simulink model "Ghost"  (Simulink 8.1)
settings: Solver=ode1  StartTime=0.0  StopTime=inf  FixedStep=Ts  MaxStep=1e-3  RelTol=1e-3
PostLoadFcn:
  | NREL_Mode=1; Ghost_init;
InitFcn:
  | NREL_Mode=1; Ghost_init;
values from neighbouring files (symbols this model uses):
  Ts = 100E-6    (= 0.0001)    [BANSHEE_init.m]    (also in Ghost_init.m)
undefined symbols (not defined in the file or in its folder): Stim
libraries: simulink x75, artemis x11, relay_housing_lib x4, rtlab x1, utility_service_lib x1, communications_lib x1, Feeder1_lib x1, Feeder2_lib x1, Feeder3_lib x1, Feeder4_lib x1, powerlib x1
(part 1 of 2)
settings Model: ARTEMISmethode_block_infos=$$__separator__$$Ghost/ARTEMIS Guide$$__separator__$$  Creator=RE25624  LastModifiedBy=pkoralew  BufferReuse=off
settings SolverCC: ZeroCrossAlgorithm=Adaptive
settings DataIOCC: ExternalInput=getinputstruct(op_snapshot1)  InitialState=getstatestruct(op_snapshot1)  LimitDataPoints=off  MaxDataPoints=90060  SignalLoggingSaveFormat=Dataset  SaveOutput=off  SignalLogging=off  DSMLogging=off  SaveTime=off  OutputSaveName=result
settings OptimizationCC: BlockReduction=off  OptimizeBlockIOStorage=off  BufferReuse=off  ExpressionFolding=off  LocalBlockOutputs=off
settings DebuggingCC: MaxConsecutiveZCsMsg=warning  IgnoredZcDiagnostic=none  SolverPrmCheckMsg=none  MultiTaskRateTransMsg=warning  ParameterPrecisionLossMsg=none  FcnCallInpInsideContextMsg=EnableAllAsWarning  FrameProcessingCompatibilityMsg=error  ModelReferenceExtraNoncontSigs=warning  StrictBusMsg=Warning
settings ModelReferenceCC: UpdateModelReferenceTargets=IfOutOfDate
settings SFSimCC: SFSimEcho=off
settings GRTTargetCC: CodeReplacementLibrary=C89/C90 (ANSI)

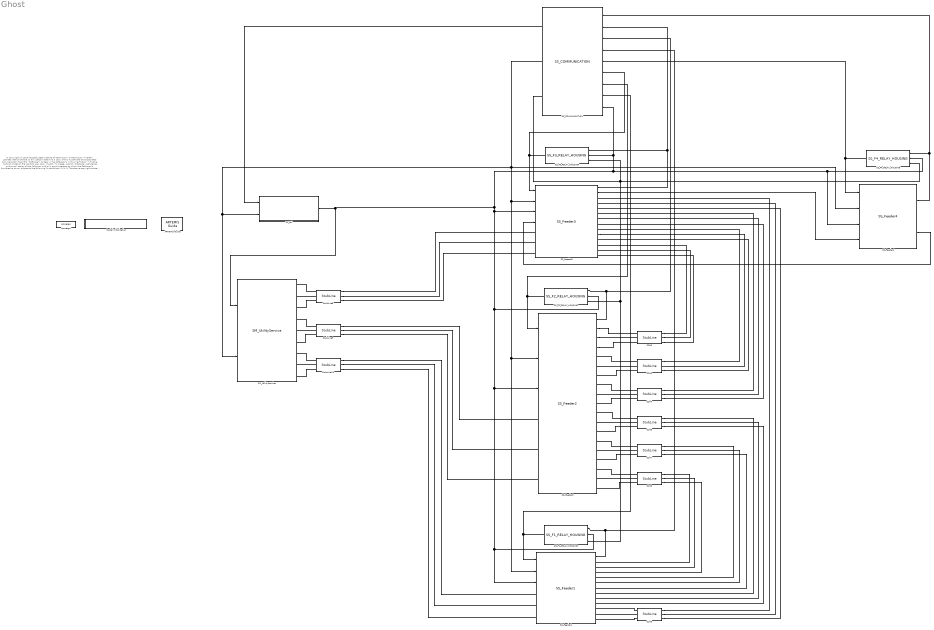
== system Ghost ==
  note: % Copyright (c) 2016 Massachusetts Institute of Technology
      | % Permission is hereby granted, free of charge, to any person obtaining a copy of this
      | % software and associated documentation files (the "Software"), to deal in the Software
      | % without restriction, including without limitation the rights to use, copy, modify,
      | % merge, publish, distribute, sublicense, and/or sell copies of the Software, and to
      | % permit persons to whom the Software is furnished to do so, subject to the following
      | % conditions:
      | %
      | %
      | % The above copyright notice and this permission notice shall be included in
      | % all copies or substantial portions of the Software.
      | %
      | % THE SOFTWARE IS PROVIDED "AS IS", WITHOUT WARRANTY OF ANY KIND, EXPRESS OR IMPLIED,
      | % INCLUDING BUT NOT LIMITED TO THE WARRANTIES OF MERCHANTABILITY, FITNESS FOR A
      | % PARTICULAR PURPOSE AND NONINFRINGEMENT. IN NO EVENT SHALL THE AUTHORS OR COPYRIGHT
      | % HOLDERS BE LIABLE FOR ANY CLAIM, DAMAGES OR OTHER LIABILITY, WHETHER IN AN ACTION
      | % OF CONTRACT, TORT OR OTHERWISE, ARISING FROM, OUT OF OR IN CONNECTION WITH THE
      | % SOFTWARE OR THE USE OR OTHER DEALINGS IN THE SOFTWARE.
      | %
      | %
      | %%
  ARTEMIS Guide : artemis/ARTEMIS/ARTEMIS Guide  Tag=FTSSmethode_opal_4hx0r99  Description=5.0_z1  lock=on  Ts=Ts  opt=art5  dyna=off  nb_perm=4  RT_fullcomp=off  ssn=on  ssn_itvc=off  ssn_ivic=off  ssn_ext=off  ssn_solver=Art5 with Backward Euler nodal interface  ssn_impulse=off  ssn_quasimpulse=off  ssn_impulse_loop=5  paraExtinctionThy=off  Thy_Impulse=on  dtc=Off  dtc_opt=normal  ao=on  simtype=off  ct_mac=off  lin_mov=off  lsp=[0.001 2]  spike_skip=Disabled  dtc_extra=1  dtc_sws=normal  dtc_pied=0.5  SPSRulesBlock=SPSRules  tre=on  ctmm=off  LF=off  dpl_type=ARTEMiS DPL  rlc_type=off  custom_type=off  para=on  ssn_ImpulseLoopBlockedStateUpdate=5  ssn_mov_iter_number=5  ssn_switch_iter_number=5  ssn_nib_type_verify=on
  C105 : artemis/ARTEMIS/StubLine  Phases=3  pu=on  L=3000 * 9.257e-08 / 1  Lpu=0.08  R=3000 * 2.94e-5 / 1  Rpu=0.002  S_base=7e6/3  V_base=13800/sqrt(3)  F_base=60  Ts=Ts
  C107 : artemis/ARTEMIS/StubLine  Phases=3  pu=on  L=2000 * 9.257e-8 / 2  Lpu=0.08  R=2000 * 2.94e-5 / 2  Rpu=0.002  S_base=4e6/3  V_base=4160/sqrt(3)  F_base=60  Ts=Ts
  C108 : artemis/ARTEMIS/StubLine  Phases=3  pu=on  L=1000 * 9.257e-8 / 2  Lpu=0.04  R=1000 * 2.94e-5 / 2  Rpu=0.002  S_base=465e3/3  V_base=480/sqrt(3)  F_base=60  Ts=Ts
  C109 : artemis/ARTEMIS/StubLine  Phases=3  pu=on  L=2000 * 9.257e-08 / 2  Lpu=0.08  R=2000 * 2.94e-5 / 2  Rpu=0.004  S_base=465e3/3  V_base=480/sqrt(3)  F_base=60  Ts=Ts
  C204 : artemis/ARTEMIS/StubLine  Phases=3  pu=on  L=1500 * 9.257e-08 / 2  Lpu=0.06  R=1500 * 2.94e-5 / 2  Rpu=0.002  S_base=465e3/3  V_base=480/sqrt(3)  F_base=60  Ts=Ts
  C205 : artemis/ARTEMIS/StubLine  Phases=3  pu=on  L=1500 * 9.257e-08 / 2  Lpu=0.06  R=1500 * 2.94e-5 / 2  Rpu=0.002  S_base=465e3/3  V_base=480/sqrt(3)  F_base=60  Ts=Ts
  C206 : artemis/ARTEMIS/StubLine  Phases=3  pu=on  L=1500 * 9.257e-08 / 2  Lpu=0.06  R=1500 * 2.94e-5 / 2  Rpu=0.002  S_base=465e3/3  V_base=480/sqrt(3)  F_base=60  Ts=Ts
  Model Initialization : Subsystem  AncestorBlock=artemis/Tools /Misc/Model Initialization  mask(Model Functions){InitFcnX=NREL_Mode=1; Ghost_init;, prel=off, posl=on, inif=on, strf=off}
      mask prompts: InitFcnX "Initialisation"; prel "Preload Function"; posl "PostLoad Function"; inif "InitFcn"; strf "StartFcn"
      mask init:
      | currentBlock = gcb;
      | root = bdroot(currentBlock);
      | 
      | if ~strcmp(get_param(root,'BlockDiagramType'),'library')
      |     if prel==1
      |         set_param(root, 'PreLoadFcn', InitFcnX);
      |     else
      |         set_param(root, 'PreLoadFcn', '');
      |     end
      |     if inif==1
      |         set_param(root, 'InitFcn', InitFcnX);
      |     else
      |         set_param(root, 'InitFcn', '');
      |     end
      |     if strf==1
      |         set_param(root, 'StartFcn', InitFcnX);
      |     else
      |         set_param(root, 'StartFcn', '');
      |     end
      |     if posl==1
      |         set_param(root, 'PostLoadFcn', InitFcnX);
      |     else
      |         set_param(root, 'PostLoadFcn', '');
      |     end
      | end
      | 
      | pos = get_param(currentBlock, 'Position');
      | width = pos(3) - pos(1); height = pos(4) - pos(2);
      | txt = [ upper(root) '\n' '- InitFcn. . . . . '  get_param(root, 'InitFcn') ];
      settings: CopyFcn=set_param(gcb,'LinkStatus','inactive')
      mask Display: text(5, height*0.5, txt, 'horizontalAlignment', 'left', 'verticalAlignment', 'middle') ;
  SC_ctrl : Subsystem
  SM_UtilityService : utility_service_lib/SM_UtilityService
  SS_COMMUNICATION : communications_lib/SS_COMMUNICATION
  SS_F1_RELAY_HOUSING : relay_housing_lib/SS_F1_RELAY_HOUSING
  SS_F2_RELAY_HOUSING : relay_housing_lib/SS_F2_RELAY_HOUSING
  SS_F3_RELAY_HOUSING : relay_housing_lib/SS_F3_RELAY_HOUSING
  SS_F4_RELAY_HOUSING : relay_housing_lib/SS_F4_RELAY_HOUSING
  SS_Feeder1 : Feeder1_lib/SS_Feeder1
  SS_Feeder2 : Feeder2_lib/SS_Feeder2
  SS_Feeder3 : Feeder3_lib/SS_Feeder3
  SS_Feeder4 : Feeder4_lib/SS_Feeder4
  StubLine10 : artemis/ARTEMIS/StubLine  Phases=3  pu=on  L=1500 * 9.43453e-08 / 2  Lpu=0.08  R=1500 * 2.28409e-5 / 2  Rpu=0.002  S_base=50e6/3  V_base=13.8e3/sqrt(3)  F_base=60  Ts=Ts
  StubLine8 : artemis/ARTEMIS/StubLine  Phases=3  pu=on  L=1500 * 9.43453e-08 / 2  Lpu=0.08  R=1500 * 2.28409e-5 / 2  Rpu=0.002  S_base=50e6/3  V_base=13.8e3/sqrt(3)  F_base=60  Ts=Ts
  StubLine9 : artemis/ARTEMIS/StubLine  Phases=3  pu=on  L=1500 * 9.43453e-08 / 2  Lpu=0.08  R=1500 * 2.28409e-5 / 2  Rpu=0.002  S_base=50e6/3  V_base=13.8e3/sqrt(3)  F_base=60  Ts=Ts
  powergui : powerlib/powergui  Priority=2  SimulationMode=Discrete  SolverType=Tustin  SampleTime=Ts  frequency=60  SPID=off  DisableSnubberDevices=off  DisableRonSwitches=off  DisableVfSwitches=off  SwTol=0  Interpol=off  DisplayEquations=off  frequencyindice=0  Pbase=100e6  ErrMax=1e-4  Iterations=50  UnitsV=kV  UnitsW=MW  FunctionMessages=off  echomessages=off  HookPort=off  EnableUseOfTLC=off  x0status=blocks  RestoreLinks=warning  ResistiveCurrentMeasurement=off  Frange=logspace(0,3,50)  Ylog=off  Xlog=off  ShowGrid=off  save=off  variable=ZData  structure=0  ZoomFFT=on  StartTime=0.0  cycles=2  DisplayStyle=off  fundamental=60  FreqAxis=off  MaxFrequency=1000  frequencyindicesteady=1  RmsSteady=1  display=off  Ts=0  methode=off
  wires:
  SS_Feeder3/1 -> SS_COMMUNICATION/2, SS_F3_RELAY_HOUSING/1
  SS_F3_RELAY_HOUSING/1 -> SS_COMMUNICATION/6, SS_Feeder3/1
  SS_F1_RELAY_HOUSING/1 -> SS_COMMUNICATION/8, SS_Feeder1/1
  SS_F2_RELAY_HOUSING/1 -> SS_COMMUNICATION/7, SS_Feeder2/1
  SS_Feeder1/1 -> SS_F1_RELAY_HOUSING/1, SS_COMMUNICATION/4
  SS_Feeder2/1 -> SS_COMMUNICATION/3, SS_F2_RELAY_HOUSING/1
  SS_COMMUNICATION/1 -> SC_ctrl/1(CMBNE_SGNLS)
  SC_ctrl/1(SC_CMD) -> SS_F2_RELAY_HOUSING/2, SS_F1_RELAY_HOUSING/2, SS_Feeder1/3, SS_Feeder2/3, SS_Feeder3/3, SS_Feeder4/3, SS_F4_RELAY_HOUSING/2, SS_COMMUNICATION/9, SS_F3_RELAY_HOUSING/2, SM_UtilityService/1
  SS_F4_RELAY_HOUSING/1 -> SS_COMMUNICATION/5, SS_Feeder4/1
  SS_Feeder4/1 -> SS_COMMUNICATION/1, SS_F4_RELAY_HOUSING/1
  SS_Feeder3/2 -> SS_Feeder4/4
  SS_Feeder4/2 -> SS_Feeder3/4
  SS_COMMUNICATION/3 -> SS_F3_RELAY_HOUSING/3, SS_F2_RELAY_HOUSING/3, SS_F1_RELAY_HOUSING/3, SS_F4_RELAY_HOUSING/3
  SS_COMMUNICATION/2 -> SS_Feeder1/2, SS_Feeder2/2, SS_Feeder3/2, SM_UtilityService/2, SC_ctrl/2(TestData), SS_Feeder4/2
  connections:
  SS_Feeder2/RConn2 -- C206/LConn2
  SS_Feeder2/RConn1 -- C206/LConn1
  SS_Feeder2/RConn3 -- C206/LConn3
  C205/LConn2 -- SS_Feeder2/RConn5
  C205/LConn3 -- SS_Feeder2/RConn6
  C205/LConn1 -- SS_Feeder2/RConn4
  C204/LConn2 -- SS_Feeder2/RConn8
  C204/LConn1 -- SS_Feeder2/RConn7
  C204/LConn3 -- SS_Feeder2/RConn9
  C108/LConn3 -- SS_Feeder2/RConn12
  C108/LConn2 -- SS_Feeder2/RConn11
  C108/LConn1 -- SS_Feeder2/RConn10
  C109/LConn3 -- SS_Feeder1/RConn12
  C109/LConn2 -- SS_Feeder1/RConn11
  C109/LConn1 -- SS_Feeder1/RConn10
  C107/LConn2 -- SS_Feeder2/RConn14
  C107/LConn1 -- SS_Feeder2/RConn13
  C107/LConn3 -- SS_Feeder2/RConn15
  C105/LConn3 -- SS_Feeder2/RConn18
  C105/LConn2 -- SS_Feeder2/RConn17
  C105/LConn1 -- SS_Feeder2/RConn16
  C105/RConn1 -- SS_Feeder1/RConn1
  C105/RConn2 -- SS_Feeder1/RConn2
  C105/RConn3 -- SS_Feeder1/RConn3
  C107/RConn1 -- SS_Feeder1/RConn4
  C107/RConn2 -- SS_Feeder1/RConn5
  C107/RConn3 -- SS_Feeder1/RConn6
  C108/RConn1 -- SS_Feeder1/RConn7
  C108/RConn2 -- SS_Feeder1/RConn8
  C108/RConn3 -- SS_Feeder1/RConn9
  C204/RConn3 -- SS_Feeder3/RConn6
  C204/RConn2 -- SS_Feeder3/RConn5
  C204/RConn1 -- SS_Feeder3/RConn4
  C205/RConn3 -- SS_Feeder3/RConn9
  C205/RConn1 -- SS_Feeder3/RConn7
  C206/RConn3 -- SS_Feeder3/RConn12
  C206/RConn2 -- SS_Feeder3/RConn11
  C206/RConn1 -- SS_Feeder3/RConn10
  C109/RConn1 -- SS_Feeder3/RConn1
  C109/RConn2 -- SS_Feeder3/RConn2
  C109/RConn3 -- SS_Feeder3/RConn3
  StubLine8/LConn1 -- SM_UtilityService/RConn1
  StubLine8/LConn2 -- SM_UtilityService/RConn2
  StubLine8/LConn3 -- SM_UtilityService/RConn3
  StubLine9/LConn2 -- SM_UtilityService/RConn5
  StubLine9/LConn3 -- SM_UtilityService/RConn6
  StubLine9/LConn1 -- SM_UtilityService/RConn4
  StubLine10/LConn2 -- SM_UtilityService/RConn8
  StubLine10/LConn3 -- SM_UtilityService/RConn9
  StubLine10/LConn1 -- SM_UtilityService/RConn7
  StubLine8/RConn3 -- SS_Feeder3/LConn3
  StubLine8/RConn2 -- SS_Feeder3/LConn2
  StubLine8/RConn1 -- SS_Feeder3/LConn1
  StubLine10/RConn1 -- SS_Feeder1/LConn1
  StubLine10/RConn2 -- SS_Feeder1/LConn2
  StubLine10/RConn3 -- SS_Feeder1/LConn3
  StubLine9/RConn1 -- SS_Feeder2/LConn1
  StubLine9/RConn2 -- SS_Feeder2/LConn2
  StubLine9/RConn3 -- SS_Feeder2/LConn3
  SS_Feeder3/RConn8 -- C205/RConn2

== system Ghost/Model Initialization ==

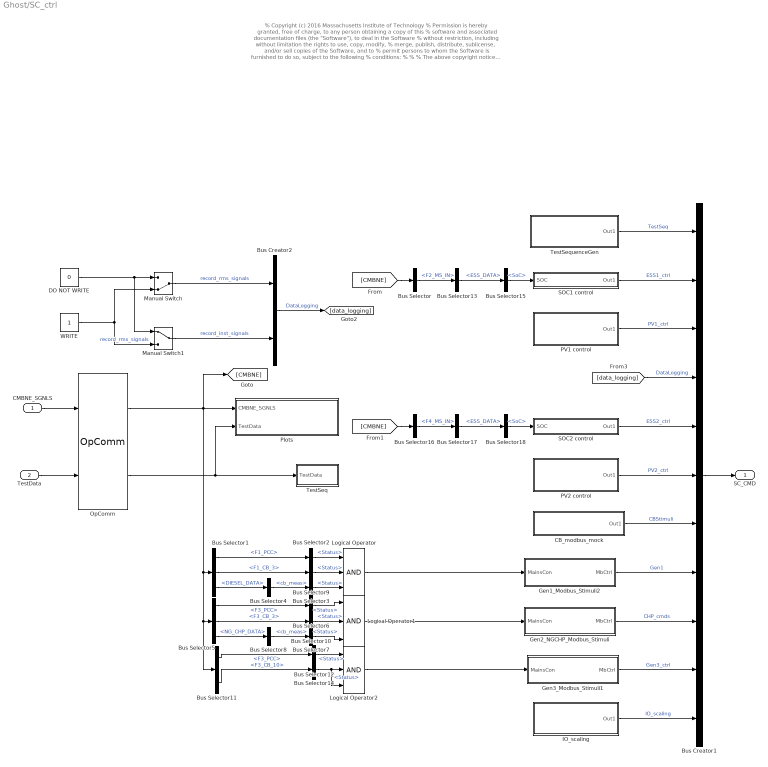
== system Ghost/SC_ctrl ==
  note: % Copyright (c) 2016 Massachusetts Institute of Technology
      | % Permission is hereby granted, free of charge, to any person obtaining a copy of this
      | % software and associated documentation files (the "Software"), to deal in the Software
      | % without restriction, including without limitation the rights to use, copy, modify,
      | % merge, publish, distribute, sublicense, and/or sell copies of the Software, and to
      | % permit persons to whom the Software is furnished to do so, subject to the following
      | % conditions:
      | %
      | %
      | % The above copyright notice and this permission notice shall be included in
      | % all copies or substantial portions of the Software.
      | %
      | % THE SOFTWARE IS PROVIDED "AS IS", WITHOUT WARRANTY OF ANY KIND, EXPRESS OR IMPLIED,
      | % INCLUDING BUT NOT LIMITED TO THE WARRANTIES OF MERCHANTABILITY, FITNESS FOR A
      | % PARTICULAR PURPOSE AND NONINFRINGEMENT. IN NO EVENT SHALL THE AUTHORS OR COPYRIGHT
      | % HOLDERS BE LIABLE FOR ANY CLAIM, DAMAGES OR OTHER LIABILITY, WHETHER IN AN ACTION
      | % OF CONTRACT, TORT OR OTHERWISE, ARISING FROM, OUT OF OR IN CONNECTION WITH THE
      | % SOFTWARE OR THE USE OR OTHER DEALINGS IN THE SOFTWARE.
      | %
      | %
      | %%
  CMBNE_SGNLS : Inport
  TestData : Inport  Port=2
  Bus Creator1 : BusCreator  Inputs=11
  Bus Creator2 : BusCreator  Inputs=2
  Bus Selector : BusSelector  OutputSignals=F2_MS_IN
  Bus Selector1 : BusSelector  OutputSignals=F1_MS_IN.CB_DATA.F1_PCC,F1_MS_IN.CB_DATA.F1_CB_3,F1_MS_IN.DIESEL_DATA
  Bus Selector{2..3,6..7,9..10,12,14} (8 alike) : BusSelector  OutputSignals=Status
  Bus Selector11 : BusSelector  OutputSignals=F3_MS_IN.CB_DATA.F3_PCC,F3_MS_IN.CB_DATA.F3_CB_10
  Bus Selector13 : BusSelector  OutputSignals=ESS_DATA
  Bus Selector15 : BusSelector  OutputSignals=Battery.SoC
  Bus Selector16 : BusSelector  OutputSignals=F4_MS_IN
  Bus Selector17 : BusSelector  OutputSignals=ESS_DATA
  Bus Selector18 : BusSelector  OutputSignals=Battery.SoC
  Bus Selector4 : BusSelector  OutputSignals=cb.cb_meas
  Bus Selector5 : BusSelector  OutputSignals=F3_MS_IN.CB_DATA.F3_PCC,F3_MS_IN.CB_DATA.F3_CB_3,F3_MS_IN.NG_CHP_DATA
  Bus Selector8 : BusSelector  OutputSignals=cb.cb_meas
  CB_modbus_mock : Subsystem
  DO NOT WRITE : Constant  Value=0
  Gen1_Modbus_Stimuli2 : Subsystem
  Gen2_NGCHP_Modbus_Stimuli : Subsystem
  Gen3_Modbus_Stimuli1 : Subsystem
  IO_scaling : Subsystem
  Logical Operator : Logic  Inputs=3  AllPortsSameDT=off  OutDataTypeStr=boolean
  Logical Operator1 : Logic  Inputs=3  AllPortsSameDT=off  OutDataTypeStr=boolean
  Logical Operator2 : Logic  Inputs=3  AllPortsSameDT=off  OutDataTypeStr=boolean
  Manual Switch : ManualSwitch  CurrentSetting=0
  Manual Switch1 : ManualSwitch
  OpComm : rtlab/OpComm  nbport=2  groupe_acq=1  subsys_rate=0  st=0  Synchronization=on  Interpolation=on  Threshold=1.0  Missed_Data=off  Sim_Time=off  Samples=off  dynSigOut=off  from_console=0  warning_done=off  writeOpCommFile=off  Offset=off
  PV1 control : Subsystem
  PV2 control : Subsystem
  Plots : Subsystem
  SOC1 control : Subsystem
  SOC2 control : Subsystem
  TestSeq : Subsystem
  TestSequenceGen : Subsystem
  WRITE : Constant
  SC_CMD : Outport
  wires:
  CMBNE_SGNLS/1 -> OpComm/1
  Bus Creator1/1 -> SC_CMD/1
  Manual Switch/1 -> Bus Creator2/1  "record_rms_signals"
  Manual Switch1/1 -> Bus Creator2/2  "record_inst_signals"
  Bus Creator2/1 -> [data_logging]  "DataLogging"
  TestData/1 -> OpComm/2
  WRITE/1 -> Manual Switch1/2, Manual Switch/2  "record_rms_signals"
  DO NOT WRITE/1 -> Manual Switch1/1, Manual Switch/1
  [data_logging] -> Bus Creator1/4  "DataLogging"
  CB_modbus_mock/1(Out1) -> Bus Creator1/7  "CBStimuli"
  Gen1_Modbus_Stimuli2/1(MbCtrl) -> Bus Creator1/8  "Gen1"
  SOC2 control/1(Out1) -> Bus Creator1/5  "ESS2_ctrl"
  PV2 control/1(Out1) -> Bus Creator1/6  "PV2_ctrl"
  Logical Operator/1 -> Gen1_Modbus_Stimuli2/1(MainsCon)
  OpComm/1 -> [CMBNE], Bus Selector11/1, Bus Selector5/1, Bus Selector1/1, Plots/1(CMBNE_SGNLS)
  Bus Selector1/1 -> Bus Selector2/1  "<F1_PCC>"
  Bus Selector1/3 -> Bus Selector4/1  "<DIESEL_DATA>"
  Bus Selector2/1 -> Logical Operator/1  "<Status>"
  Bus Selector3/1 -> Logical Operator/3  "<Status>"
  Bus Selector4/1 -> Bus Selector3/1  "<cb_meas>"
  Gen2_NGCHP_Modbus_Stimuli/1(MbCtrl) -> Bus Creator1/9  "CHP_cmds"
  Bus Selector5/1 -> Bus Selector6/1  "<F3_PCC>"
  Bus Selector5/3 -> Bus Selector8/1  "<NG_CHP_DATA>"
  Bus Selector6/1 -> Logical Operator1/1  "<Status>"
  Bus Selector7/1 -> Logical Operator1/3  "<Status>"
  Bus Selector8/1 -> Bus Selector7/1  "<cb_meas>"
  Logical Operator1/1 -> Gen2_NGCHP_Modbus_Stimuli/1(MainsCon)
  Bus Selector1/2 -> Bus Selector9/1  "<F1_CB_3>"
  Bus Selector9/1 -> Logical Operator/2  "<Status>"
  Bus Selector10/1 -> Logical Operator1/2  "<Status>"
  Bus Selector5/2 -> Bus Selector10/1  "<F3_CB_3>"
  Gen3_Modbus_Stimuli1/1(MbCtrl) -> Bus Creator1/10  "Gen3_ctrl"
  Logical Operator2/1 -> Gen3_Modbus_Stimuli1/1(MainsCon)
  Bus Selector11/1 -> Bus Selector12/1  "<F3_PCC>"
  Bus Selector12/1 -> Logical Operator2/1  "<Status>"
  Bus Selector11/2 -> Bus Selector14/1  "<F3_CB_10>"
  Bus Selector14/1 -> Logical Operator2/3, Logical Operator2/2  "<Status>"
  OpComm/2 -> Plots/2(TestData), TestSeq/1(TestData)
  IO_scaling/1(Out1) -> Bus Creator1/11  "IO_scaling"
  TestSequenceGen/1(Out1) -> Bus Creator1/1  "TestSeq"
  SOC1 control/1(Out1) -> Bus Creator1/2  "ESS1_ctrl"
  PV1 control/1(Out1) -> Bus Creator1/3  "PV1_ctrl"
  [CMBNE] -> Bus Selector/1
  Bus Selector/1 -> Bus Selector13/1  "<F2_MS_IN>"
  Bus Selector13/1 -> Bus Selector15/1  "<ESS_DATA>"
  Bus Selector15/1 -> SOC1 control/1(SOC)  "<SoC>"
  [CMBNE] -> Bus Selector16/1
  Bus Selector16/1 -> Bus Selector17/1  "<F4_MS_IN>"
  Bus Selector17/1 -> Bus Selector18/1  "<ESS_DATA>"
  Bus Selector18/1 -> SOC2 control/1(SOC)  "<SoC>"

== system Ghost/SC_ctrl/CB_modbus_mock ==
  note: Should be from pattern generator
  Bus Creator1 : BusCreator  Inputs=7
  Enabled : Constant
  F1 : Subsystem
  F2 : Subsystem
  F3 : Subsystem
  F4 : Subsystem
  Manual Switch{,1..3} (4 alike) : ManualSwitch
  Manual Switch4 : ManualSwitch  CurrentSetting=0
  NO FAULT : Constant  Value=0
  NO FAULT2 : Constant  Value=0
  NO FAULT3 : Constant  Value=0
  Pulse Generator : DiscretePulseGenerator  SampleTime=[Stim.Ts Ts]
  RST : Constant
  Rate Transition : RateTransition  Deterministic=off
  setting #1 : Constant  Value=0
  setting #2 : Constant
  Out1 : Outport
  wires:
  Bus Creator1/1 -> Rate Transition/1
  F4/1(Out1) -> Bus Creator1/4  "F4"
  F3/1(Out1) -> Bus Creator1/3  "F3"
  F2/1(Out1) -> Bus Creator1/2  "F2"
  F1/1(Out1) -> Bus Creator1/1  "F1"
  Manual Switch/1 -> Bus Creator1/5  "ResetAll"
  Manual Switch1/1 -> Manual Switch/2
  Pulse Generator/1 -> Manual Switch/1
  NO FAULT/1 -> Manual Switch1/1
  RST/1 -> Manual Switch1/2  "record_rms_signals"
  Manual Switch3/1 -> Manual Switch2/2
  NO FAULT2/1 -> Manual Switch2/1
  setting #1/1 -> Manual Switch3/1
  setting #2/1 -> Manual Switch3/2  "record_rms_signals"
  Manual Switch2/1 -> Bus Creator1/6  "GroupSel"
  Manual Switch4/1 -> Bus Creator1/7  "MockEna"
  NO FAULT3/1 -> Manual Switch4/1
  Enabled/1 -> Manual Switch4/2  "record_rms_signals"
  Rate Transition/1 -> Out1/1

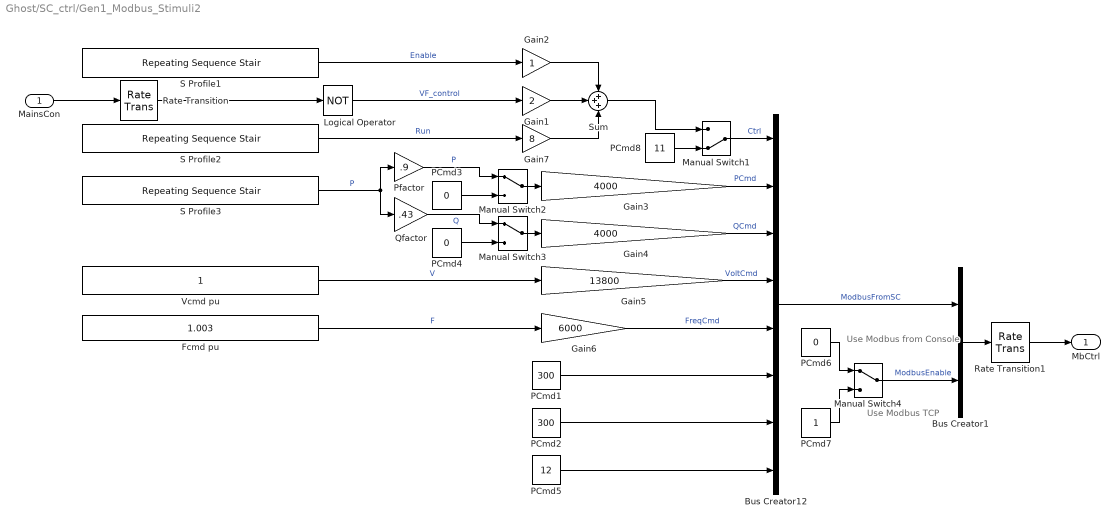
== system Ghost/SC_ctrl/Gen1_Modbus_Stimuli2 ==
  note: Use Modbus from
      | Console
  note: Use Modbus TCP
  MainsCon : Inport
  Bus Creator1 : BusCreator  Inputs=2
  Bus Creator12 : BusCreator  Inputs=8
  Fcmd pu : Constant  Value=1.003
  Gain1 : Gain  Gain=2  OutDataTypeStr=double
  Gain2 : Gain
  Gain3 : Gain  Gain=4000
  Gain4 : Gain  Gain=4000
  Gain5 : Gain  Gain=13800
  Gain6 : Gain  Gain=6000
  Gain7 : Gain  Gain=8
  Logical Operator : Logic  Operator=NOT  AllPortsSameDT=off  OutDataTypeStr=boolean
  Manual Switch1 : ManualSwitch  CurrentSetting=0
  Manual Switch2 : ManualSwitch
  Manual Switch3 : ManualSwitch
  Manual Switch4 : ManualSwitch
  PCmd1 : Constant  Value=300
  PCmd2 : Constant  Value=300
  PCmd3 : Constant  Value=0
  PCmd4 : Constant  Value=0
  PCmd5 : Constant  Value=12
  PCmd6 : Constant  Value=0
  PCmd7 : Constant
  PCmd8 : Constant  Value=11
  Pfactor : Gain  Gain=.9
  Qfactor : Gain  Gain=.43
  Rate Transition : RateTransition  Deterministic=off
  Rate Transition1 : RateTransition  Deterministic=off
  S Profile1 : simulink/Sources/Repeating Sequence Stair  OutValues=Stim.Gen3.Ena  tsamp=[Stim.Ts Ts]  OutMin=[]  OutMax=[]  OutDataTypeStr=Inherit: Inherit via back propagation  OutDataType=fixdt(0,8)  ConRadixGroup=Best Precision: Vector-wise  OutScaling=2^-12
  S Profile2 : simulink/Sources/Repeating Sequence Stair  OutValues=Stim.Gen3.Run  tsamp=[Stim.Ts Ts]  OutMin=[]  OutMax=[]  OutDataTypeStr=Inherit: Inherit via back propagation  OutDataType=fixdt(0,8)  ConRadixGroup=Best Precision: Vector-wise  OutScaling=2^-12
  S Profile3 : simulink/Sources/Repeating Sequence Stair  OutValues=Stim.Gen3.s  tsamp=[Stim.Ts Ts]  OutMin=[]  OutMax=[]  OutDataTypeStr=Inherit: Inherit via back propagation  OutDataType=fixdt(0,8)  ConRadixGroup=Best Precision: Vector-wise  OutScaling=2^-12
  Sum : Sum  Inputs=+++
  Vcmd pu : Constant
  MbCtrl : Outport
  wires:
  S Profile3/1 -> Pfactor/1, Qfactor/1  "P"
  Qfactor/1 -> Manual Switch3/1  "Q"
  Vcmd pu/1 -> Gain5/1  "V"
  Fcmd pu/1 -> Gain6/1  "F"
  Pfactor/1 -> Manual Switch2/1  "P"
  S Profile1/1 -> Gain2/1  "Enable"
  Manual Switch2/1 -> Gain3/1
  Bus Creator12/1 -> Bus Creator1/1  "ModbusFromSC"
  Manual Switch3/1 -> Gain4/1
  PCmd4/1 -> Manual Switch3/2
  PCmd3/1 -> Manual Switch2/2
  Gain2/1 -> Sum/1
  Gain1/1 -> Sum/2
  Sum/1 -> Manual Switch1/1
  PCmd1/1 -> Bus Creator12/6
  PCmd2/1 -> Bus Creator12/7
  PCmd5/1 -> Bus Creator12/8
  Bus Creator1/1 -> Rate Transition1/1
  Manual Switch4/1 -> Bus Creator1/2  "ModbusEnable"
  PCmd6/1 -> Manual Switch4/1
  PCmd7/1 -> Manual Switch4/2
  Gain3/1 -> Bus Creator12/2  "PCmd"
  Gain4/1 -> Bus Creator12/3  "QCmd"
  Gain5/1 -> Bus Creator12/4  "VoltCmd"
  Gain6/1 -> Bus Creator12/5  "FreqCmd"
  S Profile2/1 -> Gain7/1  "Run"
  Gain7/1 -> Sum/3
  MainsCon/1 -> Rate Transition/1
  Logical Operator/1 -> Gain1/1  "VF_control"
  Rate Transition/1 -> Logical Operator/1
  Rate Transition1/1 -> MbCtrl/1
  Manual Switch1/1 -> Bus Creator12/1  "Ctrl"
  PCmd8/1 -> Manual Switch1/2

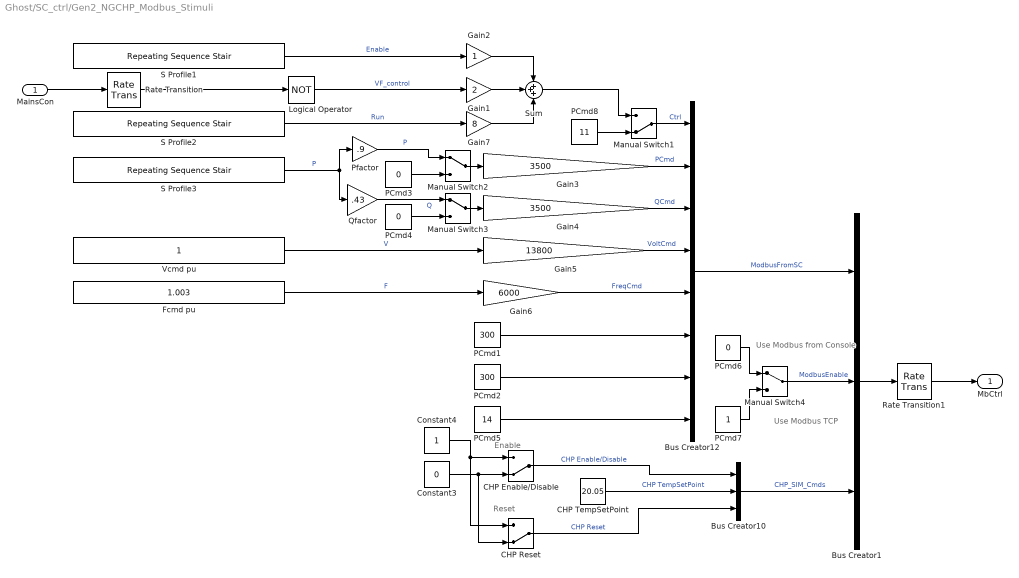
== system Ghost/SC_ctrl/Gen2_NGCHP_Modbus_Stimuli ==
  note: Use Modbus TCP
  note: Use Modbus from
      | Console
  note: Enable
  note: Reset
  MainsCon : Inport
  Bus Creator1 : BusCreator  Inputs=3
  Bus Creator10 : BusCreator  Inputs=3
  Bus Creator12 : BusCreator  Inputs=8
  CHP Enable/Disable : ManualSwitch  CurrentSetting=0
  CHP Reset : ManualSwitch  CurrentSetting=0
  CHP TempSetPoint : Constant  Value=20.05
  Constant3 : Constant  Value=0
  Constant4 : Constant
  Fcmd pu : Constant  Value=1.003
  Gain1 : Gain  Gain=2  OutDataTypeStr=double
  Gain2 : Gain
  Gain3 : Gain  Gain=3500
  Gain4 : Gain  Gain=3500
  Gain5 : Gain  Gain=13800
  Gain6 : Gain  Gain=6000
  Gain7 : Gain  Gain=8
  Logical Operator : Logic  Operator=NOT  AllPortsSameDT=off  OutDataTypeStr=boolean
  Manual Switch1 : ManualSwitch  CurrentSetting=0
  Manual Switch2 : ManualSwitch
  Manual Switch3 : ManualSwitch
  Manual Switch4 : ManualSwitch
  PCmd1 : Constant  Value=300
  PCmd2 : Constant  Value=300
  PCmd3 : Constant  Value=0
  PCmd4 : Constant  Value=0
  PCmd5 : Constant  Value=14
  PCmd6 : Constant  Value=0
  PCmd7 : Constant
  PCmd8 : Constant  Value=11
  Pfactor : Gain  Gain=.9
  Qfactor : Gain  Gain=.43
  Rate Transition : RateTransition  Deterministic=off
  Rate Transition1 : RateTransition  Deterministic=off
  S Profile1 : simulink/Sources/Repeating Sequence Stair  OutValues=Stim.Gen3.Ena  tsamp=[Stim.Ts Ts]  OutMin=[]  OutMax=[]  OutDataTypeStr=Inherit: Inherit via back propagation  OutDataType=fixdt(0,8)  ConRadixGroup=Best Precision: Vector-wise  OutScaling=2^-12
  S Profile2 : simulink/Sources/Repeating Sequence Stair  OutValues=Stim.Gen3.Run  tsamp=[Stim.Ts Ts]  OutMin=[]  OutMax=[]  OutDataTypeStr=Inherit: Inherit via back propagation  OutDataType=fixdt(0,8)  ConRadixGroup=Best Precision: Vector-wise  OutScaling=2^-12
  S Profile3 : simulink/Sources/Repeating Sequence Stair  OutValues=Stim.Gen3.s  tsamp=[Stim.Ts Ts]  OutMin=[]  OutMax=[]  OutDataTypeStr=Inherit: Inherit via back propagation  OutDataType=fixdt(0,8)  ConRadixGroup=Best Precision: Vector-wise  OutScaling=2^-12
  Sum : Sum  Inputs=+++
  Vcmd pu : Constant
  MbCtrl : Outport
  wires:
  Rate Transition/1 -> Logical Operator/1
  Logical Operator/1 -> Gain1/1  "VF_control"
  MainsCon/1 -> Rate Transition/1
  Gain7/1 -> Sum/3
  S Profile2/1 -> Gain7/1  "Run"
  Gain6/1 -> Bus Creator12/5  "FreqCmd"
  Gain5/1 -> Bus Creator12/4  "VoltCmd"
  Gain4/1 -> Bus Creator12/3  "QCmd"
  Gain3/1 -> Bus Creator12/2  "PCmd"
  PCmd7/1 -> Manual Switch4/2
  PCmd6/1 -> Manual Switch4/1
  Manual Switch4/1 -> Bus Creator1/2  "ModbusEnable"
  Bus Creator1/1 -> Rate Transition1/1
  PCmd5/1 -> Bus Creator12/8
  PCmd2/1 -> Bus Creator12/7
  PCmd1/1 -> Bus Creator12/6
  Sum/1 -> Manual Switch1/1
  Gain1/1 -> Sum/2
  Gain2/1 -> Sum/1
  PCmd3/1 -> Manual Switch2/2
  PCmd4/1 -> Manual Switch3/2
  Manual Switch3/1 -> Gain4/1
  Bus Creator12/1 -> Bus Creator1/1  "ModbusFromSC"
  Manual Switch2/1 -> Gain3/1
  S Profile1/1 -> Gain2/1  "Enable"
  Pfactor/1 -> Manual Switch2/1  "P"
  Fcmd pu/1 -> Gain6/1  "F"
  Vcmd pu/1 -> Gain5/1  "V"
  Qfactor/1 -> Manual Switch3/1  "Q"
  S Profile3/1 -> Qfactor/1, Pfactor/1  "P"
  Bus Creator10/1 -> Bus Creator1/3  "CHP_SIM_Cmds"
  CHP Reset/1 -> Bus Creator10/3  "CHP Reset"
  CHP TempSetPoint/1 -> Bus Creator10/2  "CHP TempSetPoint"
  CHP Enable/Disable/1 -> Bus Creator10/1  "CHP Enable/Disable"
  Constant4/1 -> CHP Enable/Disable/1, CHP Reset/1
  Constant3/1 -> CHP Enable/Disable/2, CHP Reset/2
  Rate Transition1/1 -> MbCtrl/1
  PCmd8/1 -> Manual Switch1/2
  Manual Switch1/1 -> Bus Creator12/1  "Ctrl"

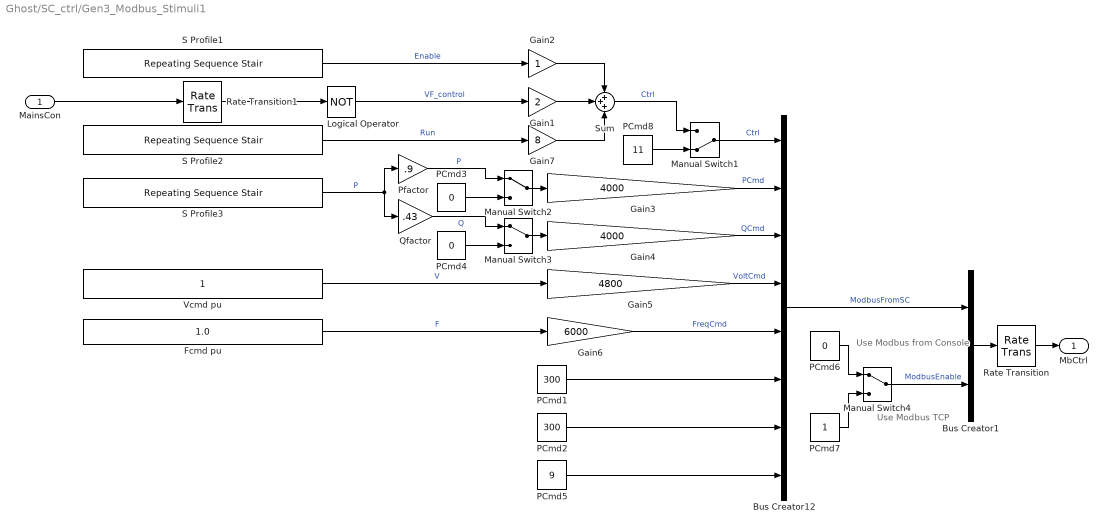
== system Ghost/SC_ctrl/Gen3_Modbus_Stimuli1 ==
  note: Use Modbus TCP
  note: Use Modbus from
      | Console
  MainsCon : Inport
  Bus Creator1 : BusCreator  Inputs=2
  Bus Creator12 : BusCreator  Inputs=8
  Fcmd pu : Constant  Value=1.0
  Gain1 : Gain  Gain=2  OutDataTypeStr=double
  Gain2 : Gain
  Gain3 : Gain  Gain=4000
  Gain4 : Gain  Gain=4000
  Gain5 : Gain  Gain=4800
  Gain6 : Gain  Gain=6000
  Gain7 : Gain  Gain=8
  Logical Operator : Logic  Operator=NOT  AllPortsSameDT=off  OutDataTypeStr=boolean
  Manual Switch1 : ManualSwitch  CurrentSetting=0
  Manual Switch2 : ManualSwitch
  Manual Switch3 : ManualSwitch
  Manual Switch4 : ManualSwitch
  PCmd1 : Constant  Value=300
  PCmd2 : Constant  Value=300
  PCmd3 : Constant  Value=0
  PCmd4 : Constant  Value=0
  PCmd5 : Constant  Value=9
  PCmd6 : Constant  Value=0
  PCmd7 : Constant
  PCmd8 : Constant  Value=11
  Pfactor : Gain  Gain=.9
  Qfactor : Gain  Gain=.43
  Rate Transition : RateTransition  Deterministic=off
  Rate Transition1 : RateTransition  Deterministic=off
  S Profile1 : simulink/Sources/Repeating Sequence Stair  OutValues=Stim.Gen3.Ena  tsamp=[Stim.Ts Ts]  OutMin=[]  OutMax=[]  OutDataTypeStr=Inherit: Inherit via back propagation  OutDataType=fixdt(0,8)  ConRadixGroup=Best Precision: Vector-wise  OutScaling=2^-12
  S Profile2 : simulink/Sources/Repeating Sequence Stair  OutValues=Stim.Gen3.Run  tsamp=[Stim.Ts Ts]  OutMin=[]  OutMax=[]  OutDataTypeStr=Inherit: Inherit via back propagation  OutDataType=fixdt(0,8)  ConRadixGroup=Best Precision: Vector-wise  OutScaling=2^-12
  S Profile3 : simulink/Sources/Repeating Sequence Stair  OutValues=Stim.Gen3.s  tsamp=[Stim.Ts Ts]  OutMin=[]  OutMax=[]  OutDataTypeStr=Inherit: Inherit via back propagation  OutDataType=fixdt(0,8)  ConRadixGroup=Best Precision: Vector-wise  OutScaling=2^-12
  Sum : Sum  Inputs=+++
  Vcmd pu : Constant
  MbCtrl : Outport
  wires:
  MainsCon/1 -> Rate Transition1/1
  Logical Operator/1 -> Gain1/1  "VF_control"
  Gain7/1 -> Sum/3
  S Profile2/1 -> Gain7/1  "Run"
  Gain6/1 -> Bus Creator12/5  "FreqCmd"
  Gain5/1 -> Bus Creator12/4  "VoltCmd"
  Gain4/1 -> Bus Creator12/3  "QCmd"
  Gain3/1 -> Bus Creator12/2  "PCmd"
  PCmd7/1 -> Manual Switch4/2
  PCmd6/1 -> Manual Switch4/1
  Manual Switch4/1 -> Bus Creator1/2  "ModbusEnable"
  Bus Creator1/1 -> Rate Transition/1
  PCmd5/1 -> Bus Creator12/8
  PCmd2/1 -> Bus Creator12/7
  PCmd1/1 -> Bus Creator12/6
  Sum/1 -> Manual Switch1/1  "Ctrl"
  Gain1/1 -> Sum/2
  Gain2/1 -> Sum/1
  PCmd3/1 -> Manual Switch2/2
  PCmd4/1 -> Manual Switch3/2
  Manual Switch3/1 -> Gain4/1
  Bus Creator12/1 -> Bus Creator1/1  "ModbusFromSC"
  Manual Switch2/1 -> Gain3/1
  S Profile1/1 -> Gain2/1  "Enable"
  Pfactor/1 -> Manual Switch2/1  "P"
  Fcmd pu/1 -> Gain6/1  "F"
  Vcmd pu/1 -> Gain5/1  "V"
  Qfactor/1 -> Manual Switch3/1  "Q"
  S Profile3/1 -> Qfactor/1, Pfactor/1  "P"
  Rate Transition/1 -> MbCtrl/1
  Rate Transition1/1 -> Logical Operator/1
  PCmd8/1 -> Manual Switch1/2
  Manual Switch1/1 -> Bus Creator12/1  "Ctrl"

== system Ghost/SC_ctrl/IO_scaling ==
  Bus Creator12 : BusCreator  Inputs=11
  Manual Switch : ManualSwitch
  PCmd1 : Constant  Value=1.015
  PCmd10 : Constant  Value=[1.1 0.8]
  PCmd2 : Constant  Value=[ 6 6 6 ]
  PCmd{3,6,8..9} (4 alike) : Constant
  PCmd4 : Constant  Value=125
  PCmd5 : Constant  Value=6
  PCmd7 : Constant  Value=10/600
  Real_measurements : Constant
  Sim_measurements : Constant  Value=0
  Out1 : Outport
  wires:
  PCmd7/1 -> Bus Creator12/3  "AOUT_I_GAIN"
  Bus Creator12/1 -> Out1/1
  PCmd6/1 -> Bus Creator12/2  "AIN_I_GAIN"
  PCmd3/1 -> Bus Creator12/1  "AIN_V_GAIN"
  PCmd1/1 -> Bus Creator12/4  "AOUT_V_GAIN"
  Manual Switch/1 -> Bus Creator12/5  "PHIL_Enabled"
  Real_measurements/1 -> Manual Switch/2  "record_rms_signals"
  Sim_measurements/1 -> Manual Switch/1
  PCmd4/1 -> Bus Creator12/6  "I_sense_gain"
  PCmd5/1 -> Bus Creator12/7  "I_sense_offset"
  PCmd2/1 -> Bus Creator12/8  "I_gen_offset"
  PCmd9/1 -> Bus Creator12/9  "V_dq_mode_ena"
  PCmd10/1 -> Bus Creator12/10  "V_mag_limits"
  PCmd8/1 -> Bus Creator12/11  "Vang_enable"

== system Ghost/SC_ctrl/PV1 control ==
  note: Use Modbus TCP
  note: Use Modbus from
      | Console
  Bus Creator1 : BusCreator  Inputs=3
  Bus Creator12 : BusCreator  Inputs=8
  Gain3 : Gain  Gain=5000
  Gain4 : Gain  Gain=5000
  Gain5 : Gain  Gain=4800
  Gain6 : Gain  Gain=6000
  Manual Switch : ManualSwitch  CurrentSetting=0
  Manual Switch1 : ManualSwitch  CurrentSetting=0
  Manual Switch2 : ManualSwitch
  Manual Switch3 : ManualSwitch  CurrentSetting=0
  PCmd{1..2,4,6} (4 alike) : Constant  Value=0
  PCmd3 : Constant  Value=0.7
  PCmd5 : Constant  Value=11
  PCmd7 : Constant
  PCmd8 : Constant
  Rate Transition : RateTransition  Deterministic=off
  S Profile1 : simulink/Sources/Repeating Sequence Stair  OutValues=Stim.PV2.Ena  tsamp=[Stim.Ts Ts]  OutMin=[]  OutMax=[]  OutDataTypeStr=Inherit: Inherit via back propagation  OutDataType=fixdt(0,8)  ConRadixGroup=Best Precision: Vector-wise  OutScaling=2^-12
  S Profile2 : simulink/Sources/Repeating Sequence Stair  OutValues=Stim.ESS2.p  tsamp=[Stim.Ts Ts]  OutMin=[]  OutMax=[]  OutDataTypeStr=Inherit: Inherit via back propagation  OutDataType=fixdt(0,8)  ConRadixGroup=Best Precision: Vector-wise  OutScaling=2^-12
  S Profile3 : simulink/Sources/Repeating Sequence Stair  OutValues=Stim.ESS2.q  tsamp=[Stim.Ts Ts]  OutMin=[]  OutMax=[]  OutDataTypeStr=Inherit: Inherit via back propagation  OutDataType=fixdt(0,8)  ConRadixGroup=Best Precision: Vector-wise  OutScaling=2^-12
  S Profile4 : simulink/Sources/Repeating Sequence Stair  OutValues=Stim.ESS2.v  tsamp=[Stim.Ts Ts]  OutMin=[]  OutMax=[]  OutDataTypeStr=Inherit: Inherit via back propagation  OutDataType=fixdt(0,8)  ConRadixGroup=Best Precision: Vector-wise  OutScaling=2^-12
  S Profile5 : simulink/Sources/Repeating Sequence Stair  OutValues=Stim.ESS2.f  tsamp=[Stim.Ts Ts]  OutMin=[]  OutMax=[]  OutDataTypeStr=Inherit: Inherit via back propagation  OutDataType=fixdt(0,8)  ConRadixGroup=Best Precision: Vector-wise  OutScaling=2^-12
  Tuning : Subsystem
  Out1 : Outport
  wires:
  Rate Transition/1 -> Out1/1
  Gain6/1 -> Bus Creator12/5  "FreqCmd"
  Gain5/1 -> Bus Creator12/4  "VoltCmd"
  Gain4/1 -> Bus Creator12/3  "QCmd"
  Gain3/1 -> Bus Creator12/2  "PCmd"
  PCmd7/1 -> Manual Switch2/2
  PCmd6/1 -> Manual Switch2/1
  Manual Switch2/1 -> Bus Creator1/2  "ModbusEnable"
  Bus Creator1/1 -> Rate Transition/1
  PCmd5/1 -> Bus Creator12/8
  PCmd2/1 -> Bus Creator12/7
  PCmd1/1 -> Bus Creator12/6
  S Profile1/1 -> Manual Switch3/1
  S Profile3/1 -> Manual Switch1/1
  S Profile2/1 -> Manual Switch/1
  PCmd3/1 -> Manual Switch/2
  PCmd4/1 -> Manual Switch1/2
  S Profile4/1 -> Gain5/1
  Manual Switch1/1 -> Gain4/1
  Bus Creator12/1 -> Bus Creator1/1  "ModbusFromSC"
  Manual Switch/1 -> Gain3/1
  S Profile5/1 -> Gain6/1
  PCmd8/1 -> Manual Switch3/2
  Manual Switch3/1 -> Bus Creator12/1  "Ctrl"
  Tuning/1(Tuning) -> Bus Creator1/3  "Tuning"

== system Ghost/SC_ctrl/PV2 control ==
  note: Use Modbus from
      | Console
  note: Use Modbus TCP
  Bus Creator1 : BusCreator  Inputs=3
  Bus Creator12 : BusCreator  Inputs=8
  Gain3 : Gain  Gain=1000
  Gain4 : Gain  Gain=1000
  Gain5 : Gain  Gain=4800
  Gain6 : Gain  Gain=6000
  Manual Switch : ManualSwitch  CurrentSetting=0
  Manual Switch1 : ManualSwitch  CurrentSetting=0
  Manual Switch2 : ManualSwitch
  Manual Switch3 : ManualSwitch  CurrentSetting=0
  PCmd{1..2,4,6} (4 alike) : Constant  Value=0
  PCmd3 : Constant
  PCmd5 : Constant  Value=11
  PCmd7 : Constant
  PCmd8 : Constant
  Rate Transition : RateTransition  Deterministic=off
  S Profile1 : simulink/Sources/Repeating Sequence Stair  OutValues=Stim.PV2.Ena  tsamp=[Stim.Ts Ts]  OutMin=[]  OutMax=[]  OutDataTypeStr=Inherit: Inherit via back propagation  OutDataType=fixdt(0,8)  ConRadixGroup=Best Precision: Vector-wise  OutScaling=2^-12
  S Profile2 : simulink/Sources/Repeating Sequence Stair  OutValues=Stim.ESS2.p  tsamp=[Stim.Ts Ts]  OutMin=[]  OutMax=[]  OutDataTypeStr=Inherit: Inherit via back propagation  OutDataType=fixdt(0,8)  ConRadixGroup=Best Precision: Vector-wise  OutScaling=2^-12
  S Profile3 : simulink/Sources/Repeating Sequence Stair  OutValues=Stim.ESS2.q  tsamp=[Stim.Ts Ts]  OutMin=[]  OutMax=[]  OutDataTypeStr=Inherit: Inherit via back propagation  OutDataType=fixdt(0,8)  ConRadixGroup=Best Precision: Vector-wise  OutScaling=2^-12
  S Profile4 : simulink/Sources/Repeating Sequence Stair  OutValues=Stim.ESS2.v  tsamp=[Stim.Ts Ts]  OutMin=[]  OutMax=[]  OutDataTypeStr=Inherit: Inherit via back propagation  OutDataType=fixdt(0,8)  ConRadixGroup=Best Precision: Vector-wise  OutScaling=2^-12
  S Profile5 : simulink/Sources/Repeating Sequence Stair  OutValues=Stim.ESS2.f  tsamp=[Stim.Ts Ts]  OutMin=[]  OutMax=[]  OutDataTypeStr=Inherit: Inherit via back propagation  OutDataType=fixdt(0,8)  ConRadixGroup=Best Precision: Vector-wise  OutScaling=2^-12
  Tuning : Subsystem
  Out1 : Outport
  wires:
  Manual Switch3/1 -> Bus Creator12/1  "Ctrl"
  PCmd8/1 -> Manual Switch3/2
  S Profile5/1 -> Gain6/1
  Manual Switch/1 -> Gain3/1
  Bus Creator12/1 -> Bus Creator1/1  "ModbusFromSC"
  Manual Switch1/1 -> Gain4/1
  S Profile4/1 -> Gain5/1
  PCmd4/1 -> Manual Switch1/2
  PCmd3/1 -> Manual Switch/2
  S Profile2/1 -> Manual Switch/1
  S Profile3/1 -> Manual Switch1/1
  S Profile1/1 -> Manual Switch3/1
  PCmd1/1 -> Bus Creator12/6
  PCmd2/1 -> Bus Creator12/7
  PCmd5/1 -> Bus Creator12/8
  Bus Creator1/1 -> Rate Transition/1
  Manual Switch2/1 -> Bus Creator1/2  "ModbusEnable"
  PCmd6/1 -> Manual Switch2/1
  PCmd7/1 -> Manual Switch2/2
  Gain3/1 -> Bus Creator12/2  "PCmd"
  Gain4/1 -> Bus Creator12/3  "QCmd"
  Gain5/1 -> Bus Creator12/4  "VoltCmd"
  Gain6/1 -> Bus Creator12/5  "FreqCmd"
  Rate Transition/1 -> Out1/1
  Tuning/1(Tuning) -> Bus Creator1/3  "Tuning"

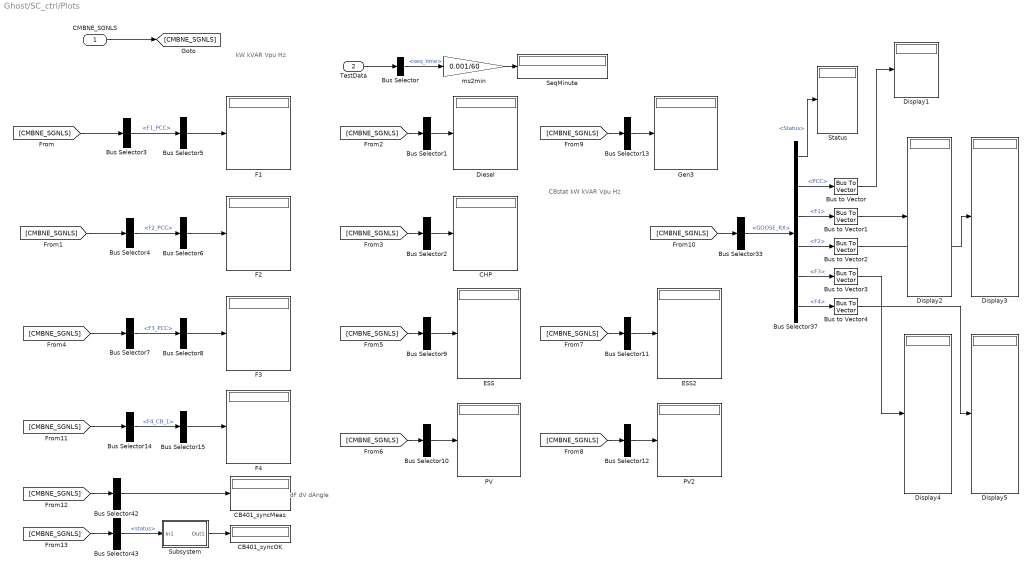
== system Ghost/SC_ctrl/Plots ==
  note: kW
      | kVAR
      | Vpu
      | Hz
  note: CBstat
      | kW
      | kVAR
      | Vpu
      | Hz
  note: dF
      | dV
      | dAngle
  CMBNE_SGNLS : Inport
  TestData : Inport  Port=2
  Bus Selector : BusSelector  OutputSignals=TestSeq.seq_time
  Bus Selector1 : BusSelector  OutputSignals=F1_MS_IN.DIESEL_DATA.cb.cb_meas.Status,F1_MS_IN.DIESEL_DATA.cb.relay_out.m.kw,F1_MS_IN.DIESEL_DATA.cb.relay_out.m.kvar,F1_MS_IN.DIESEL_DATA.cb.relay_out.m.Va_rms,F1_MS_IN.DIESEL_DATA.cb.relay_out.m.Hz  OutputAsBus=on
  Bus Selector10 : BusSelector  OutputSignals=F2_MS_IN.PV_DATA.CB_meas.cb_meas.Status,F2_MS_IN.PV_DATA.CB_meas.relay_out.m.kw,F2_MS_IN.PV_DATA.CB_meas.relay_out.m.kvar,F2_MS_IN.PV_DATA.CB_meas.relay_out.m.Va_rms,F2_MS_IN.PV_DATA.CB_meas.relay_out.m.Hz  OutputAsBus=on
  Bus Selector11 : BusSelector  OutputSignals=F4_MS_IN.ESS_DATA.CB_meas.cb_meas.Status,F4_MS_IN.ESS_DATA.CB_meas.relay_out.m.kw,F4_MS_IN.ESS_DATA.CB_meas.relay_out.m.kvar,F4_MS_IN.ESS_DATA.CB_meas.relay_out.m.Va_rms,F4_MS_IN.ESS_DATA.CB_meas.relay_out.m.Hz,F4_MS_IN.ESS_DATA.Battery.SoC  OutputAsBus=on
  Bus Selector12 : BusSelector  OutputSignals=F4_MS_IN.PV_DATA.CB_meas.cb_meas.Status,F4_MS_IN.PV_DATA.CB_meas.relay_out.m.kw,F4_MS_IN.PV_DATA.CB_meas.relay_out.m.kvar,F4_MS_IN.PV_DATA.CB_meas.relay_out.m.Va_rms,F4_MS_IN.PV_DATA.CB_meas.relay_out.m.Hz  OutputAsBus=on
  Bus Selector13 : BusSelector  OutputSignals=F4_MS_IN.GEN3_DATA.cb.cb_meas.Status,F4_MS_IN.GEN3_DATA.cb.relay_out.m.kw,F4_MS_IN.GEN3_DATA.cb.relay_out.m.kvar,F4_MS_IN.GEN3_DATA.cb.relay_out.m.Va_rms,F4_MS_IN.GEN3_DATA.cb.relay_out.m.Hz  OutputAsBus=on
  Bus Selector14 : BusSelector  OutputSignals=F4_RELAY_OUT.F4_CB_1
  Bus Selector{5..6,8,15} (4 alike) : BusSelector  OutputSignals=m.kw,m.kvar,m.Vpu,m.Hz  OutputAsBus=on
  Bus Selector2 : BusSelector  OutputSignals=F3_MS_IN.NG_CHP_DATA.cb.cb_meas.Status,F3_MS_IN.NG_CHP_DATA.cb.relay_out.m.kw,F3_MS_IN.NG_CHP_DATA.cb.relay_out.m.kvar,F3_MS_IN.NG_CHP_DATA.cb.relay_out.m.Va_rms,F3_MS_IN.NG_CHP_DATA.cb.relay_out.m.Hz  OutputAsBus=on
  Bus Selector3 : BusSelector  OutputSignals=F1_RELAY_OUT.F1_PCC
  Bus Selector33 : BusSelector  OutputSignals=GOOSE_RX
  Bus Selector37 : BusSelector  OutputSignals=Status,PCC,F1,F2,F3,F4
  Bus Selector4 : BusSelector  OutputSignals=F2_RELAY_OUT.F2_PCC
  Bus Selector42 : BusSelector  OutputSignals=F4_RELAY_OUT.cb401_syncMeas.dF,F4_RELAY_OUT.cb401_syncMeas.dV,F4_RELAY_OUT.cb401_syncMeas.dWt  OutputAsBus=on
  Bus Selector43 : BusSelector  OutputSignals=F4_RELAY_OUT.F4_CB_1.m.status
  Bus Selector7 : BusSelector  OutputSignals=F3_RELAY_OUT.F3_PCC
  Bus Selector9 : BusSelector  OutputSignals=F2_MS_IN.ESS_DATA.CB_meas.cb_meas.Status,F2_MS_IN.ESS_DATA.CB_meas.relay_out.m.kw,F2_MS_IN.ESS_DATA.CB_meas.relay_out.m.kvar,F2_MS_IN.ESS_DATA.CB_meas.relay_out.m.Va_rms,F2_MS_IN.ESS_DATA.CB_meas.relay_out.m.Hz,F2_MS_IN.ESS_DATA.Battery.SoC  OutputAsBus=on
  Bus to Vector{,1..4} (5 alike) : BusToVector
  CB401_syncMeas : Display
  CB401_syncOK : Display
  CHP : Display
  Diesel : Display
  Display{1..5} (5 alike) : Display
  ESS : Display
  ESS2 : Display
  F{1..4} (4 alike) : Display
  Gen3 : Display
  PV : Display
  PV2 : Display
  SeqMinute : Display
  Status : Display
  Subsystem : Subsystem
  ms2min : Gain  Gain=0.001/60
  wires:
  Bus Selector5/1 -> F1/1
  Bus Selector4/1 -> Bus Selector6/1  "<F2_PCC>"
  Bus Selector1/1 -> Diesel/1
  Bus Selector2/1 -> CHP/1
  CMBNE_SGNLS/1 -> [CMBNE_SGNLS]
  [CMBNE_SGNLS] -> Bus Selector3/1
  [CMBNE_SGNLS] -> Bus Selector4/1
  [CMBNE_SGNLS] -> Bus Selector7/1
  [CMBNE_SGNLS] -> Bus Selector2/1
  [CMBNE_SGNLS] -> Bus Selector1/1
  Bus Selector3/1 -> Bus Selector5/1  "<F1_PCC>"
  Bus Selector7/1 -> Bus Selector8/1  "<F3_PCC>"
  Bus Selector9/1 -> ESS/1
  [CMBNE_SGNLS] -> Bus Selector9/1
  Bus Selector10/1 -> PV/1
  [CMBNE_SGNLS] -> Bus Selector10/1
  Bus Selector11/1 -> ESS2/1
  [CMBNE_SGNLS] -> Bus Selector11/1
  Bus Selector12/1 -> PV2/1
  [CMBNE_SGNLS] -> Bus Selector12/1
  Bus Selector13/1 -> Gen3/1
  [CMBNE_SGNLS] -> Bus Selector13/1
  [CMBNE_SGNLS] -> Bus Selector33/1
  Bus Selector33/1 -> Bus Selector37/1  "<GOOSE_RX>"
  Bus Selector37/1 -> Status/1  "<Status>"
  Bus Selector37/2 -> Bus to Vector/1  "<PCC>"
  Bus to Vector/1 -> Display1/1
  Bus Selector37/3 -> Bus to Vector1/1  "<F1>"
  Bus Selector37/6 -> Bus to Vector4/1  "<F4>"
  Bus Selector37/5 -> Bus to Vector3/1  "<F3>"
  Bus Selector37/4 -> Bus to Vector2/1  "<F2>"
  Bus to Vector4/1 -> Display5/1
  Bus to Vector3/1 -> Display4/1
  Bus to Vector2/1 -> Display3/1
  Bus to Vector1/1 -> Display2/1
  Bus Selector/1 -> ms2min/1  "<seq_time>"
  TestData/1 -> Bus Selector/1
  ms2min/1 -> SeqMinute/1
  [CMBNE_SGNLS] -> Bus Selector14/1
  Bus Selector14/1 -> Bus Selector15/1  "<F4_CB_1>"
  Bus Selector6/1 -> F2/1
  Bus Selector15/1 -> F4/1
  Bus Selector8/1 -> F3/1
  Bus Selector42/1 -> CB401_syncMeas/1
  [CMBNE_SGNLS] -> Bus Selector42/1
  [CMBNE_SGNLS] -> Bus Selector43/1
  Bus Selector43/1 -> Subsystem/1(In1)  "<status>"
  Subsystem/1(Out1) -> CB401_syncOK/1

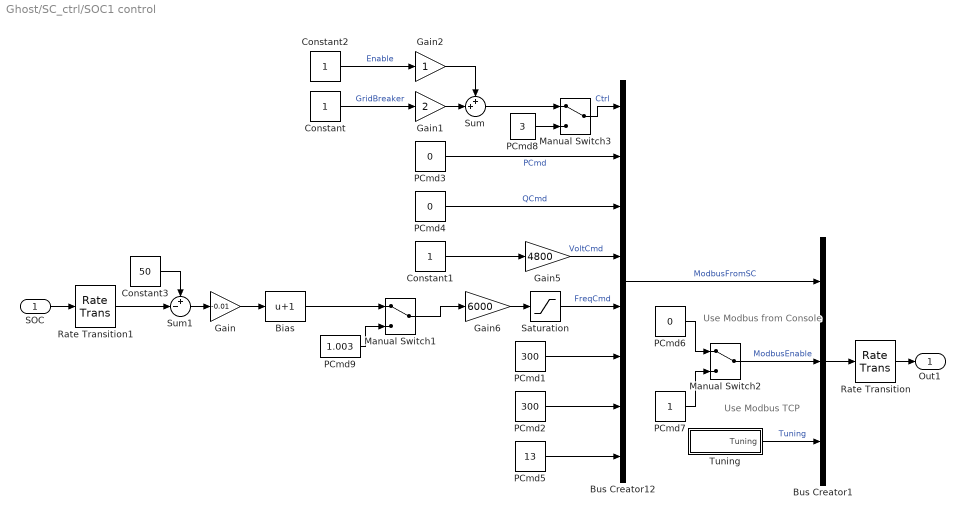
== system Ghost/SC_ctrl/SOC1 control ==
  note: Use Modbus TCP
  note: Use Modbus from
      | Console
  SOC : Inport
  Bias : Bias  Bias=1
  Bus Creator1 : BusCreator  Inputs=3
  Bus Creator12 : BusCreator  Inputs=8
  Constant : Constant
  Constant1 : Constant
  Constant2 : Constant
  Constant3 : Constant  Value=50
  Gain : Gain  Gain=-0.01
  Gain1 : Gain  Gain=2
  Gain2 : Gain
  Gain5 : Gain  Gain=4800
  Gain6 : Gain  Gain=6000
  Manual Switch1 : ManualSwitch
  Manual Switch2 : ManualSwitch
  Manual Switch3 : ManualSwitch
  PCmd1 : Constant  Value=300
  PCmd2 : Constant  Value=300
  PCmd3 : Constant  Value=0
  PCmd4 : Constant  Value=0
  PCmd5 : Constant  Value=13
  PCmd6 : Constant  Value=0
  PCmd7 : Constant
  PCmd8 : Constant  Value=3
  PCmd9 : Constant  Value=1.003
  Rate Transition : RateTransition  Deterministic=off
  Rate Transition1 : RateTransition  Deterministic=off  OutPortSampleTime=100e-3
  Saturation : Saturate  UpperLimit=6045  LowerLimit=5955
  Sum : Sum  Inputs=++|
  Sum1 : Sum  Inputs=+-|
  Tuning : Subsystem
  Out1 : Outport
  wires:
  PCmd8/1 -> Manual Switch3/2
  Manual Switch3/1 -> Bus Creator12/1  "Ctrl"
  Gain6/1 -> Saturation/1
  Gain5/1 -> Bus Creator12/4  "VoltCmd"
  PCmd4/1 -> Bus Creator12/3  "QCmd"
  PCmd3/1 -> Bus Creator12/2  "PCmd"
  PCmd7/1 -> Manual Switch2/2
  PCmd6/1 -> Manual Switch2/1
  Manual Switch2/1 -> Bus Creator1/2  "ModbusEnable"
  Bus Creator1/1 -> Rate Transition/1
  PCmd5/1 -> Bus Creator12/8
  PCmd2/1 -> Bus Creator12/7
  PCmd1/1 -> Bus Creator12/6
  Sum/1 -> Manual Switch3/1
  Gain1/1 -> Sum/2
  Gain2/1 -> Sum/1
  Constant1/1 -> Gain5/1
  Constant2/1 -> Gain2/1  "Enable"
  Bus Creator12/1 -> Bus Creator1/1  "ModbusFromSC"
  Constant/1 -> Gain1/1  "GridBreaker"
  Rate Transition/1 -> Out1/1
  Saturation/1 -> Bus Creator12/5  "FreqCmd"
  Bias/1 -> Manual Switch1/1
  Constant3/1 -> Sum1/1
  SOC/1 -> Rate Transition1/1
  Sum1/1 -> Gain/1
  Gain/1 -> Bias/1
  Rate Transition1/1 -> Sum1/2
  Manual Switch1/1 -> Gain6/1
  PCmd9/1 -> Manual Switch1/2
  Tuning/1(Tuning) -> Bus Creator1/3  "Tuning"

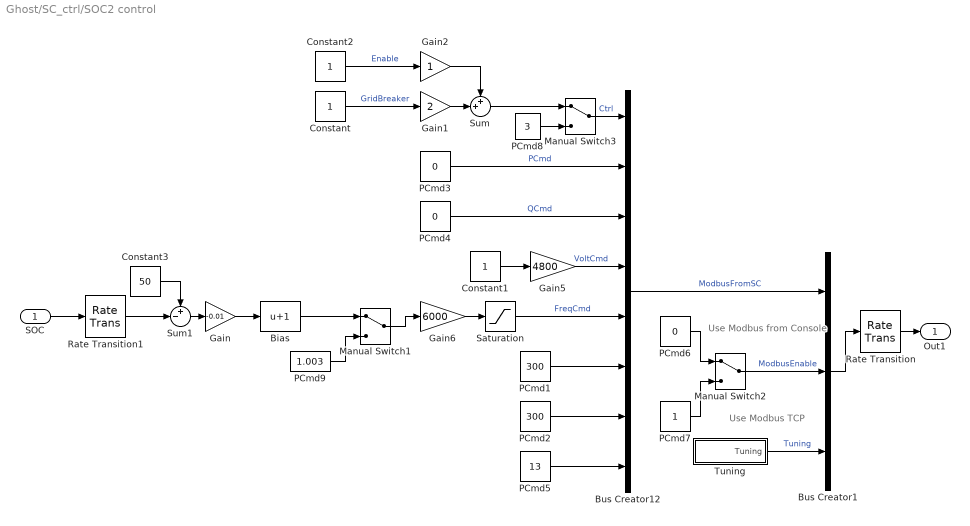
== system Ghost/SC_ctrl/SOC2 control ==
  note: Use Modbus from
      | Console
  note: Use Modbus TCP
  SOC : Inport
  Bias : Bias  Bias=1
  Bus Creator1 : BusCreator  Inputs=3
  Bus Creator12 : BusCreator  Inputs=8
  Constant : Constant
  Constant1 : Constant
  Constant2 : Constant
  Constant3 : Constant  Value=50
  Gain : Gain  Gain=-0.01
  Gain1 : Gain  Gain=2
  Gain2 : Gain
  Gain5 : Gain  Gain=4800
  Gain6 : Gain  Gain=6000
  Manual Switch1 : ManualSwitch
  Manual Switch2 : ManualSwitch
  Manual Switch3 : ManualSwitch
  PCmd1 : Constant  Value=300
  PCmd2 : Constant  Value=300
  PCmd3 : Constant  Value=0
  PCmd4 : Constant  Value=0
  PCmd5 : Constant  Value=13
  PCmd6 : Constant  Value=0
  PCmd7 : Constant
  PCmd8 : Constant  Value=3
  PCmd9 : Constant  Value=1.003
  Rate Transition : RateTransition  Deterministic=off
  Rate Transition1 : RateTransition  Deterministic=off  OutPortSampleTime=100e-3
  Saturation : Saturate  UpperLimit=6045  LowerLimit=5955
  Sum : Sum  Inputs=++|
  Sum1 : Sum  Inputs=+-|
  Tuning : Subsystem
  Out1 : Outport
  wires:
  Sum1/1 -> Gain/1
  SOC/1 -> Rate Transition1/1
  Constant3/1 -> Sum1/1
  Bias/1 -> Manual Switch1/1
  Saturation/1 -> Bus Creator12/5  "FreqCmd"
  Rate Transition/1 -> Out1/1
  Constant/1 -> Gain1/1  "GridBreaker"
  Bus Creator12/1 -> Bus Creator1/1  "ModbusFromSC"
  Constant2/1 -> Gain2/1  "Enable"
  Constant1/1 -> Gain5/1
  Gain2/1 -> Sum/1
  Gain1/1 -> Sum/2
  Sum/1 -> Manual Switch3/1
  PCmd1/1 -> Bus Creator12/6
  PCmd2/1 -> Bus Creator12/7
  PCmd5/1 -> Bus Creator12/8
  Bus Creator1/1 -> Rate Transition/1
  Manual Switch2/1 -> Bus Creator1/2  "ModbusEnable"
  PCmd6/1 -> Manual Switch2/1
  PCmd7/1 -> Manual Switch2/2
  PCmd3/1 -> Bus Creator12/2  "PCmd"
  PCmd4/1 -> Bus Creator12/3  "QCmd"
  Gain5/1 -> Bus Creator12/4  "VoltCmd"
  Gain6/1 -> Saturation/1
  Manual Switch3/1 -> Bus Creator12/1  "Ctrl"
  PCmd8/1 -> Manual Switch3/2
  Gain/1 -> Bias/1
  Rate Transition1/1 -> Sum1/2
  Manual Switch1/1 -> Gain6/1
  PCmd9/1 -> Manual Switch1/2
  Tuning/1(Tuning) -> Bus Creator1/3  "Tuning"

== system Ghost/SC_ctrl/TestSeq ==
  TestData : Inport
  Bias : Bias  Bias=[0:-1:-10]*1.1
  Bias1 : Bias  Bias=[0:-1:-2]*1.1
  Bias2 : Bias  Bias=[0:-1:-1]*1.1
  Bias3 : Bias  Bias=[0:-1:-1]*1.1
  Bus Selector : BusSelector  OutputSignals=TestSeq.seq_time,TestSeq.fault,TestSeq.dms,TestSeq.grid,TestSeq.motor,TestSeq.misc
  Bus Selector1 : BusSelector  OutputSignals=loc1,loc2,loc3,loc4,loc5,loc6,gen1,gen2,gen3,pv1,pv2  OutputAsBus=on
  Bus Selector2 : BusSelector  OutputSignals=DisReq,kWEna,PFEna  OutputAsBus=on
  Bus Selector3 : BusSelector  OutputSignals=kWref,PFref
  Bus Selector4 : BusSelector  OutputSignals=Dp,Dq  OutputAsBus=on
  Bus Selector5 : BusSelector  OutputSignals=Hz,Volt  OutputAsBus=on
  Bus Selector6 : BusSelector  OutputSignals=ena1,ena2  OutputAsBus=on
  Bus Selector7 : BusSelector  OutputSignals=cut_grid,mgc_ena  OutputAsBus=on
  Bus Selector8 : BusSelector  OutputSignals=TestSeq.price,TestSeq.pv.insolation1,TestSeq.pv.insolation2  OutputAsBus=on
  Gain : Gain  Gain=[1/60 1/115000]
  SeqMinute : Display
  TestSequence : Scope  NumInputPorts=9
      settings: YMin=-5~-5~-5~-5~-5~-5~-5~-5~-5  YMax=5~5~5~5~5~5~5~5~5  Decimation=50
  ms2min : Gain  Gain=0.001/60
  wires:
  Bus Selector8/1 -> TestSequence/9  "price, pv1, pv2"
  Bias3/1 -> TestSequence/8  "misc: cut_grid, mgc_ena"
  Bus Selector7/1 -> Bias3/1
  Bus Selector/6 -> Bus Selector7/1  "<misc>"
  Bias2/1 -> TestSequence/7  "motor: ena1, ena2"
  Bus Selector6/1 -> Bias2/1
  Bus Selector/5 -> Bus Selector6/1  "<motor>"
  Gain/1 -> TestSequence/6  "GridPU: Hz/Volt"
  Bus Selector5/1 -> Gain/1
  Bus Selector/4 -> Bus Selector5/1  "<grid>"
  Bus Selector/3 -> Bus Selector2/1, Bus Selector4/1, Bus Selector3/1  "<dms>"
  Bus Selector4/1 -> TestSequence/5  "Dp, Dq"
  Bus Selector3/2 -> TestSequence/4  "<PFref>"
  Bus Selector3/1 -> TestSequence/3  "<kWref>"
  Bias1/1 -> TestSequence/2  "dms: DisReq, kwCmd, PFCmd"
  Bus Selector2/1 -> Bias1/1
  Bias/1 -> TestSequence/1  "flt: loc1-6, gen1-3, ess1-2, pv1-2"
  Bus Selector1/1 -> Bias/1
  Bus Selector/2 -> Bus Selector1/1  "<fault>"
  Bus Selector/1 -> ms2min/1  "<seq_time>"
  TestData/1 -> Bus Selector/1, Bus Selector8/1
  ms2min/1 -> SeqMinute/1
